simulink model "chap12_1sim"  (Simulink 8.1)
settings: Solver=ode4  SolverMode=SingleTasking  StartTime=0.0  StopTime=10  FixedStep=0.001  RelTol=1e-3
settings Model: Creator=ljk  LastModifiedBy=liujk  ExtModeTrigMode=oneshot  ExtModeArmWhenConnect=off
settings DataIOCC: LimitDataPoints=off
settings OptimizationCC: BlockReduction=off  BooleanDataType=off
settings DebuggingCC: SaveWithParameterizedLinksMsg=none  SignalResolutionControl=TryResolveAllWithWarning  SolverPrmCheckMsg=none  MultiTaskDSMMsg=warning  MultiTaskCondExecSysMsg=none  StrictBusMsg=None
settings HardwareCC: TargetUnknown=on
settings RTWCC: IncludeERTFirstTime=on

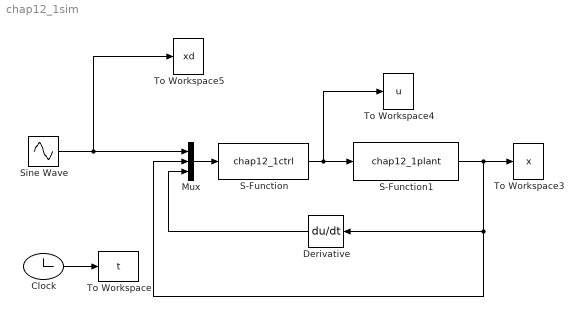
== system chap12_1sim ==
  Clock : Clock
  Derivative : Derivative
  Mux : Mux  Inputs=3
  S-Function : S-Function  FunctionName=chap12_1ctrl  EnableBusSupport=off
  S-Function1 : S-Function  FunctionName=chap12_1plant  EnableBusSupport=off
  Sine Wave : Sin  SampleTime=0
  To Workspace : ToWorkspace  VariableName=t  SampleTime=-1
  To Workspace3 : ToWorkspace  VariableName=x  SampleTime=-1
  To Workspace4 : ToWorkspace  VariableName=u  SampleTime=-1
  To Workspace5 : ToWorkspace  VariableName=xd  SampleTime=-1
  wires:
  Mux/1 -> S-Function/1
  S-Function1/1 -> To Workspace3/1, Mux/2, Derivative/1
  Clock/1 -> To Workspace/1
  S-Function/1 -> S-Function1/1, To Workspace4/1
  Derivative/1 -> Mux/3
  Sine Wave/1 -> Mux/1, To Workspace5/1
